simulink model "FMCW_Radar_1D"  (R2025b)
settings: Solver=ode4  StartTime=0.0  StopTime=0.1  FixedStep=2.5e-05  RelTol=1e-3
libraries: simulink x1
settings Model: Creator=kimsteph  LastModifiedBy=kimsteph

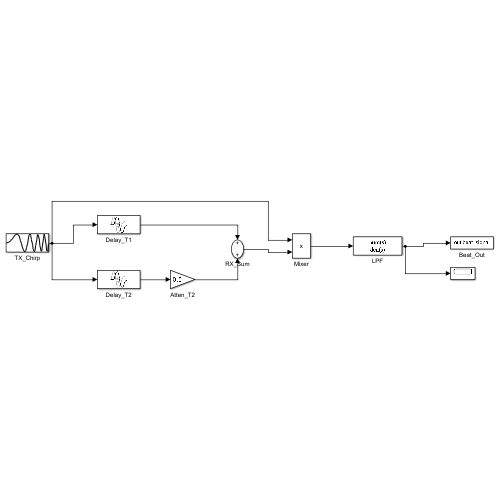
[thumbnail: Simulink's stored preview of the top-level diagram]
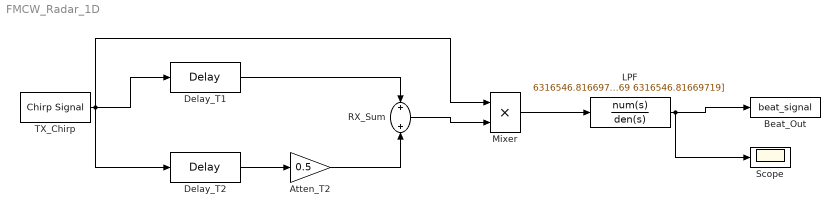
== system FMCW_Radar_1D ==
  Atten_T2 : Gain  Gain=0.5
  Beat_Out : ToWorkspace  VariableName=beat_signal  SaveFormat=Timeseries  SampleTime=-1
  Delay_T1 : TransportDelay  DelayTime=0.003
  Delay_T2 : TransportDelay  DelayTime=0.008
  LPF : TransferFcn  Numerator=6316546.81669719  Denominator=[1 3554.30635052669 6316546.81669719]
  Mixer : Product
  RX_Sum : Sum
  Scope : Scope
  TX_Chirp : simulink/Sources/Chirp Signal  f1=0  T=0.1  f2=2000
  wires:
  TX_Chirp/1 -> Delay_T1/1, Delay_T2/1, Mixer/1
  Delay_T1/1 -> RX_Sum/1
  Delay_T2/1 -> Atten_T2/1
  Atten_T2/1 -> RX_Sum/2
  RX_Sum/1 -> Mixer/2
  Mixer/1 -> LPF/1
  LPF/1 -> Beat_Out/1, Scope/1
